simulink model "Action"  (R2024b)
settings: Solver=VariableStepAuto  StartTime=0.0  StopTime=10.0  RelTol=1e-3
libraries: simulink x2
settings Model: Creator=Ahmad  LastModifiedBy=Ahmad

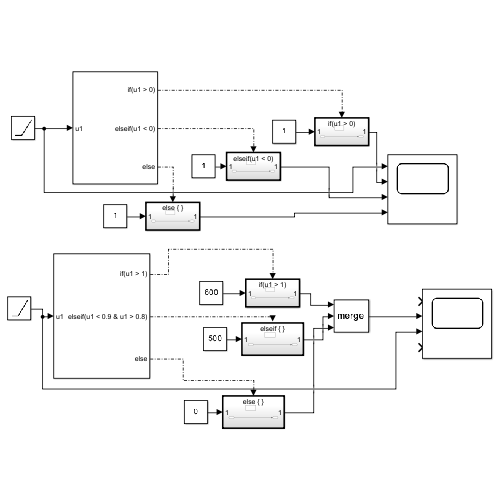
[thumbnail: Simulink's stored preview of the top-level diagram]
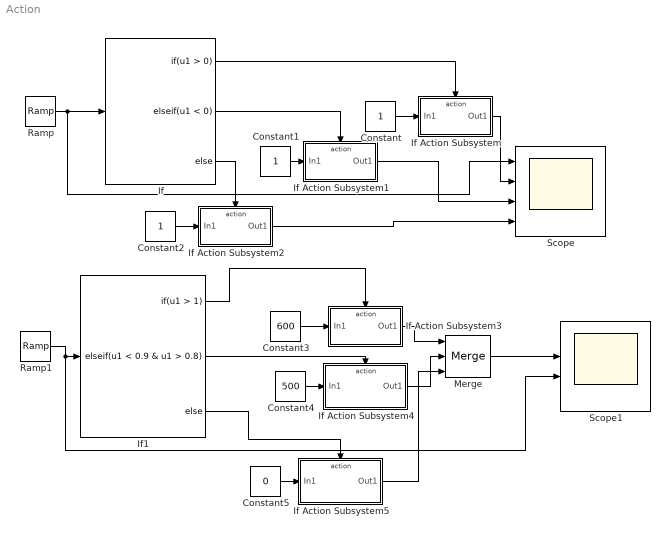
== system Action ==
  Constant : Constant
  Constant1 : Constant
  Constant2 : Constant
  Constant3 : Constant  Value=600
  Constant4 : Constant  Value=500
  Constant5 : Constant  Value=0
  If : If  ElseIfExpressions=u1 < 0
  If Action Subsystem : Subsystem  TreatAsAtomicUnit=on
  If Action Subsystem1 : Subsystem  TreatAsAtomicUnit=on
  If Action Subsystem2 : Subsystem  TreatAsAtomicUnit=on
  If Action Subsystem3 : Subsystem  TreatAsAtomicUnit=on
  If Action Subsystem4 : Subsystem  TreatAsAtomicUnit=on
  If Action Subsystem5 : Subsystem  TreatAsAtomicUnit=on
  If1 : If  IfExpression=u1 > 1  ElseIfExpressions=u1 < 0.9 & u1 > 0.8
  Merge : Merge  Inputs=3
  Ramp : simulink/Sources/Ramp  slope=1  start=1  InitialOutput=-0
  Ramp1 : simulink/Sources/Ramp  slope=1  start=1  InitialOutput=-0
  Scope : Scope  NumInputPorts=4
  Scope1 : Scope  NumInputPorts=4
  wires:
  Ramp/1 -> Scope/1, If/1
  If/1 -> If Action Subsystem/Action
  If/2 -> If Action Subsystem1/Action
  If/3 -> If Action Subsystem2/Action
  Constant/1 -> If Action Subsystem/1(In1)
  Constant1/1 -> If Action Subsystem1/1(In1)
  Constant2/1 -> If Action Subsystem2/1(In1)
  If Action Subsystem/1(Out1) -> Scope/2
  If Action Subsystem1/1(Out1) -> Scope/3
  If Action Subsystem2/1(Out1) -> Scope/4
  Constant3/1 -> If Action Subsystem3/1(In1)
  If1/1 -> If Action Subsystem3/Action
  Constant4/1 -> If Action Subsystem4/1(In1)
  If1/2 -> If Action Subsystem4/Action
  Constant5/1 -> If Action Subsystem5/1(In1)
  If1/3 -> If Action Subsystem5/Action
  Ramp1/1 -> Scope1/3, If1/1
  If Action Subsystem3/1(Out1) -> Merge/1
  If Action Subsystem4/1(Out1) -> Merge/2
  If Action Subsystem5/1(Out1) -> Merge/3
  Merge/1 -> Scope1/2

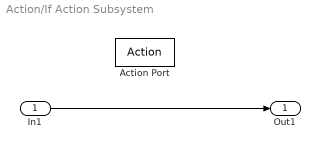
== system Action/If Action Subsystem ==
  In1 : Inport
  Action Port : ActionPort  ActionPortLabel=if(u1 > 0)
  Out1 : Outport
  wires:
  In1/1 -> Out1/1

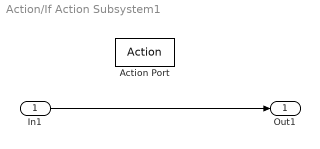
== system Action/If Action Subsystem1 ==
  In1 : Inport
  Action Port : ActionPort  ActionPortLabel=elseif(u1 < 0)
  Out1 : Outport
  wires:
  In1/1 -> Out1/1

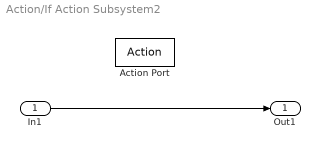
== system Action/If Action Subsystem2 ==
  In1 : Inport
  Action Port : ActionPort  ActionPortLabel=else
  Out1 : Outport
  wires:
  In1/1 -> Out1/1

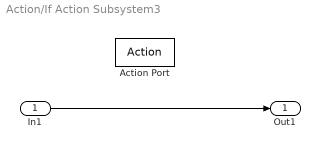
== system Action/If Action Subsystem3 ==
  In1 : Inport
  Action Port : ActionPort  ActionPortLabel=if(u1 > 1)
  Out1 : Outport
  wires:
  In1/1 -> Out1/1

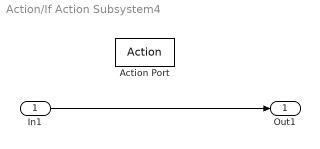
== system Action/If Action Subsystem4 ==
  In1 : Inport
  Action Port : ActionPort  ActionPortLabel=elseif(u1 < 0.9 & u1 > 0.8)
  Out1 : Outport
  wires:
  In1/1 -> Out1/1

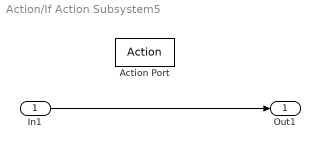
== system Action/If Action Subsystem5 ==
  In1 : Inport
  Action Port : ActionPort  ActionPortLabel=else
  Out1 : Outport
  wires:
  In1/1 -> Out1/1
